simulink model "controlloreGMV1"  (R2024b)
settings: Solver=VariableStepAuto  StartTime=0.0  StopTime=10.0  RelTol=1e-3
values from neighbouring files (symbols this model uses):
  A = media*ones(2001, 1)    [Codice.m]    (also in creAB.m = mdiagonal(A,[0 1;a1(i) a2(i)]))
  B = mdiagonal(B,[0;b1(i)])    [creAB.m]
undefined symbols (not defined in the file or in its folder): Gz
libraries: cstblocks x3
settings Model: Creator=User  LastModifiedBy=User

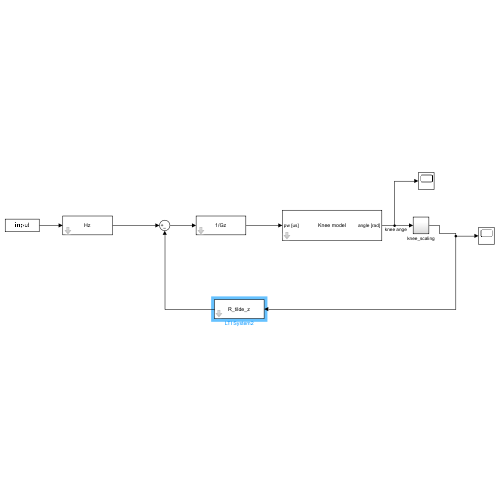
[thumbnail: Simulink's stored preview of the top-level diagram]
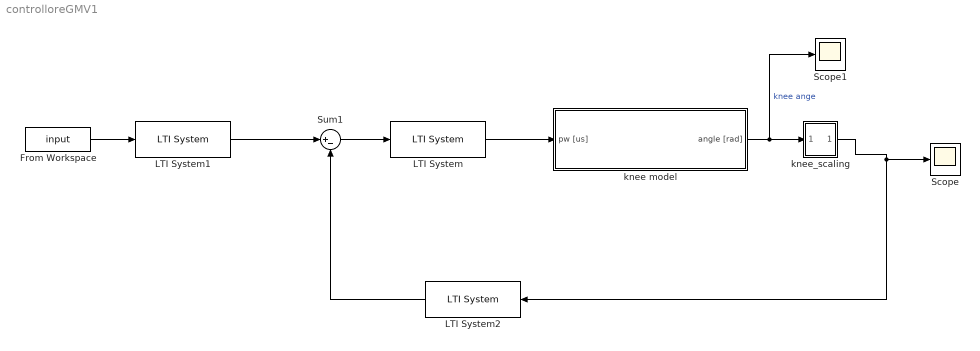
== system controlloreGMV1 ==
  From Workspace : FromWorkspace  VariableName=input
  LTI System : cstblocks/LTI System  sys=1/Gz  IC=[]  PadeOrder=0
  LTI System1 : cstblocks/LTI System  sys=Hz  IC=[]  PadeOrder=0
  LTI System2 : cstblocks/LTI System  sys=R_tilde_z  IC=[]  PadeOrder=0
  Scope : Scope
  Scope1 : Scope
  Sum1 : Sum  Inputs=|+-
  knee model : Subsystem  mask{freq=20, qk0=1.54248, act0=[0 0 0 0 0 0    0 0 0.0 0 0.0 0   0 0 0 0 0 0 ]}
      mask prompts: freq "frequency:"; qk0 "initial knee angle:"; act0 "initial states for musle activation:"
      mask init:
      | [A,B]=creAB;
      mask Display: disp('Knee model')
  knee_scaling : Subsystem
  wires:
  Sum1/1 -> LTI System/1
  From Workspace/1 -> LTI System1/1
  knee model/1(angle [rad]) -> Scope1/1, knee_scaling/1(in_1)  "knee ange"
  knee_scaling/1(knee_angle_[deg]) -> Scope/1, LTI System2/1
  LTI System/1 -> knee model/1(pw [us])
  LTI System1/1 -> Sum1/1
  LTI System2/1 -> Sum1/2

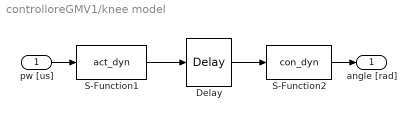
== system controlloreGMV1/knee model ==
  pw [us] : Inport
  Delay : TransportDelay  DelayTime=0.025  InitialOutput=act0(1:2:17)
  S-Function1 : S-Function  FunctionName=act_dyn  Parameters=act0,freq,A,B  SFunctionDeploymentMode=off  EnableBusSupport=off
  S-Function2 : S-Function  FunctionName=con_dyn  Parameters=qk0  SFunctionDeploymentMode=off  EnableBusSupport=off
  angle [rad] : Outport  InitialOutput=0
  wires:
  S-Function1/1 -> Delay/1
  pw [us]/1 -> S-Function1/1
  S-Function2/1 -> angle [rad]/1
  Delay/1 -> S-Function2/1

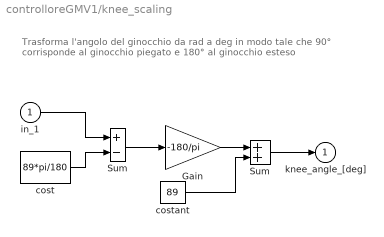
== system controlloreGMV1/knee_scaling ==
  note: Trasforma l'angolo del ginocchio da rad a deg in modo tale che
      | 90° corrisponde al ginocchio piegato e 180° al ginocchio esteso
  in_1 : Inport
  Gain : Gain  Gain=-180/pi  SaturateOnIntegerOverflow=on  OutDataTypeStr=Inherit: Same as input  ParamDataTypeStr=Inherit: Same as input
  "Sum " : Sum  Inputs=+-  InputSameDT=on  SaturateOnIntegerOverflow=on  OutDataTypeStr=Inherit: Same as first input
  "Sum " : Sum  InputSameDT=on  SaturateOnIntegerOverflow=on  OutDataTypeStr=Inherit: Same as first input
  cost : Constant  Value=89*pi/180
  "costant " : Constant  Value=89
  knee_angle_[deg] : Outport  InitialOutput=0
  wires:
  "Sum "/1 -> knee_angle_[deg]/1
  in_1/1 -> "Sum "/1
  cost/1 -> "Sum "/2
  "Sum "/1 -> Gain/1
  Gain/1 -> "Sum "/1
  "costant "/1 -> "Sum "/2
